simulink model "lab3_simple1"  (R2018a)
settings: Solver=ode45  StartTime=0.0  StopTime=10.0  RelTol=1e-3  EnableMultiTasking=on
libraries: simulink x1, truetime x1
settings Model: ExtModeAutoUpdateStatusClock=off  Creator=anton  LastModifiedBy=Ismael
settings DataIOCC: LimitDataPoints=on  SaveFormat=Array  SignalLoggingSaveFormat=ModelDataLogs
settings OptimizationCC: BooleanDataType=off  LifeSpan=inf
settings DebuggingCC: SaveWithParameterizedLinksMsg=none  UnderspecifiedInitializationDetection=Classic  MergeDetectMultiDrivingBlocksExec=none  SignalResolutionControl=TryResolveAllWithWarning  MultiTaskDSMMsg=warning  MultiTaskCondExecSysMsg=none  FcnCallInpInsideContextMsg=warning  SFUnexpectedBacktrackingDiag=warning  SFNoUnconditionalDefaultTransitionDiag=warning  SFExecutionAtInitializationDiag=none
settings HardwareCC: ProdBitPerPointer=32  ProdBitPerSizeT=32  ProdBitPerPtrDiffT=32  ProdLargestAtomicFloat=None  ProdIntDivRoundTo=Undefined  ProdEndianess=Unspecified  ProdWordSize=32  ProdHWDeviceType=32-bit Generic  TargetUnknown=on
settings ModelReferenceCC: PropagateSignalLabelsOutOfModel=off
settings CodeAppCC: StateflowObjectComments=on
settings GRTTargetCC: TargetLangStandard=C89/C90 (ANSI)  GeneratePreprocessorConditionals=Disable all  CombineOutputUpdateFcns=off  GRTInterface=on
settings ConfigComp: CovMetricSettings=dw  CovHtmlReporting=on  CovSaveCumulativeToWorkspaceVar=on  CovSaveSingleToWorkspaceVar=on  CovExternalEMLEnable=off

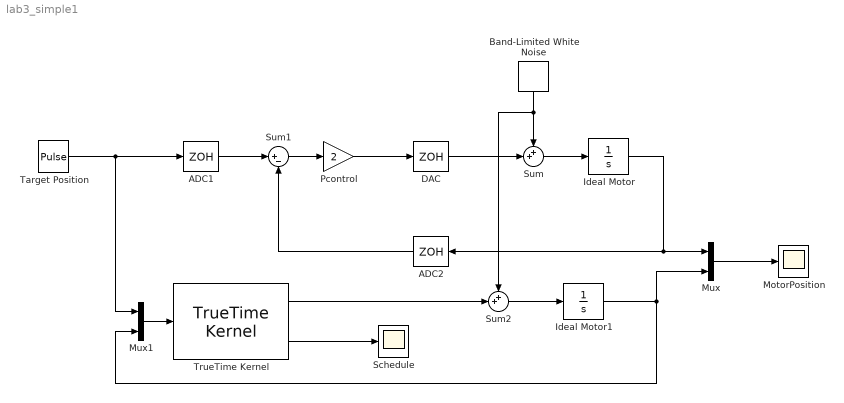
== system lab3_simple1 ==
  ADC1 : ZeroOrderHold  SampleTime=-1
  ADC2 : ZeroOrderHold  SampleTime=-1
  Band-Limited White Noise : simulink/Sources/Band-Limited White Noise  Cov=[0.1]  Ts=0.5  seed=[23341]
  DAC : ZeroOrderHold  SampleTime=-1
  Ideal Motor : Integrator
  Ideal Motor1 : Integrator
  MotorPosition : Scope
  Mux : Mux  Inputs=2
  Mux1 : Mux  Inputs=2
  Pcontrol : Gain  Gain=2
  Schedule : Scope
  Sum : Sum  Inputs=++|  SaturateOnIntegerOverflow=on  InputSameDT=on  OutDataTypeStr=Inherit: Same as first input
  Sum1 : Sum  Inputs=|+-  SaturateOnIntegerOverflow=on  InputSameDT=on  OutDataTypeStr=Inherit: Same as first input
  Sum2 : Sum  Inputs=++|  SaturateOnIntegerOverflow=on  InputSameDT=on  OutDataTypeStr=Inherit: Same as first input
  Target Position : DiscretePulseGenerator  PulseType=Time based  Period=5  PulseWidth=50
  TrueTime Kernel : truetime/TrueTime Kernel  sfun=simple_init  args=0.5  ninputsoutputs=[2 1]  ntriggers=0  trigtype=falling  nwnodenbr=[]  clockoffsetdrift=[0 0]  schedoutput=on  battery=off  poweroutput=off
  wires:
  Ideal Motor/1 -> Mux/1, ADC2/1
  Sum/1 -> Ideal Motor/1
  Band-Limited White Noise/1 -> Sum2/1, Sum/1
  Target Position/1 -> Mux1/1, ADC1/1
  ADC1/1 -> Sum1/1
  Sum1/1 -> Pcontrol/1
  Pcontrol/1 -> DAC/1
  DAC/1 -> Sum/2
  ADC2/1 -> Sum1/2
  TrueTime Kernel/2 -> Schedule/1
  Mux1/1 -> TrueTime Kernel/1
  Mux/1 -> MotorPosition/1
  TrueTime Kernel/1 -> Sum2/2
  Sum2/1 -> Ideal Motor1/1
  Ideal Motor1/1 -> Mux1/2, Mux/2
